simulink model "DC_motor"  (R2023b)
settings: Solver=VariableStepAuto  StartTime=0.0  StopTime=10.0  RelTol=1e-3
settings Model: Creator=alalar1  LastModifiedBy=alalar1

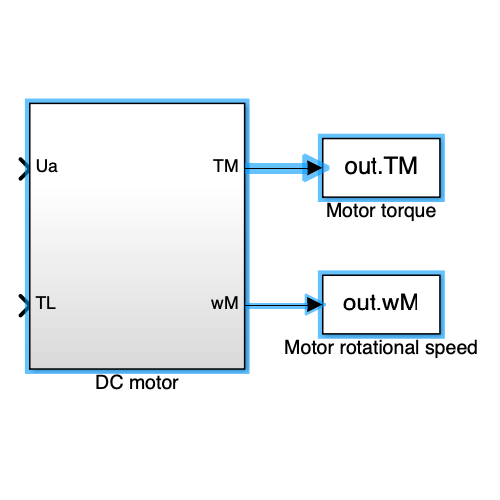
[thumbnail: Simulink's stored preview of the top-level diagram]
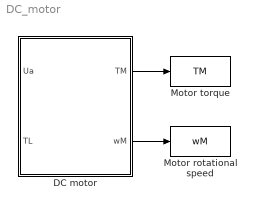
== system DC_motor ==
  DC motor : Subsystem
  Motor rotational speed : ToWorkspace  VariableName=wM  SaveFormat=Timeseries  SampleTime=-1
  Motor torque : ToWorkspace  VariableName=TM  SaveFormat=Timeseries  SampleTime=-1
  wires:
  DC motor/2(wM) -> Motor rotational speed/1
  DC motor/1(TM) -> Motor torque/1

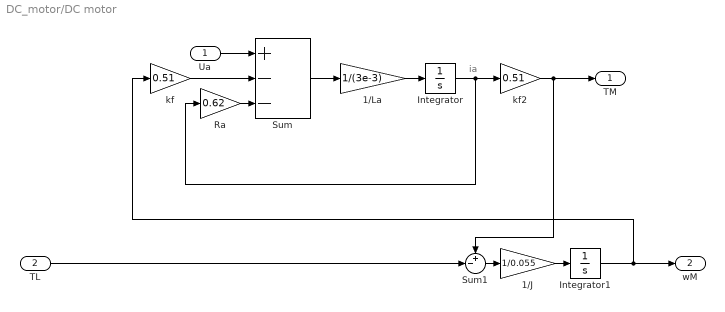
== system DC_motor/DC motor ==
  note: ia
  Ua : Inport
  TL : Inport  Port=2
  1/J : Gain  Gain=1/0.055
  1/La : Gain  Gain=1/(3e-3)
  Integrator : Integrator
  Integrator1 : Integrator
  Ra : Gain  Gain=0.62
  Sum : Sum  Inputs=+--
  Sum1 : Sum  Inputs=+-|
  kf : Gain  Gain=0.51
  kf2 : Gain  Gain=0.51
  TM : Outport  VectorParamsAs1DForOutWhenUnconnected=off
  wM : Outport  Port=2  VectorParamsAs1DForOutWhenUnconnected=off
  wires:
  Integrator/1 -> Ra/1, kf2/1
  kf2/1 -> TM/1, Sum1/1
  1/La/1 -> Integrator/1
  Sum/1 -> 1/La/1
  Ua/1 -> Sum/1
  Ra/1 -> Sum/3
  kf/1 -> Sum/2
  Integrator1/1 -> wM/1, kf/1
  1/J/1 -> Integrator1/1
  Sum1/1 -> 1/J/1
  TL/1 -> Sum1/2
